simulink model "Reg_Adapt_c"  (R2017a)
settings: Solver=ode1  StartTime=0.0  StopTime=10  FixedStep=0.0001  RelTol=1e-3
values from neighbouring files (symbols this model uses):
  gamma = 0.005    [Dane_reg_adapt.m]
  Kd1 = 0.09    [Dane_reg_adapt.m]
  Ki1 = 350    [Dane_reg_adapt.m]
  Kp1 = 7    [Dane_reg_adapt.m]
  ksi = 0.9    [Dane_reg_adapt.m]
  omega = 40    [Dane_reg_adapt.m]
  Te = 0.001    [Dane_reg_adapt.m]
  Tm = 0.2    [Dane_reg_adapt.m]
  W1init = -1*0.1    (= -0.1)    [Dane_reg_adapt.m]
  W2init = 0.2    [Dane_reg_adapt.m]
  W3init = 0.3    [Dane_reg_adapt.m]
  W4init = -1*0.4    (= -0.4)    [Dane_reg_adapt.m]
  W5init = -1*0.5    (= -0.5)    [Dane_reg_adapt.m]
  W6init = 0.6    [Dane_reg_adapt.m]
libraries: neural x6
settings Model: Creator=kamil  LastModifiedBy=kamil

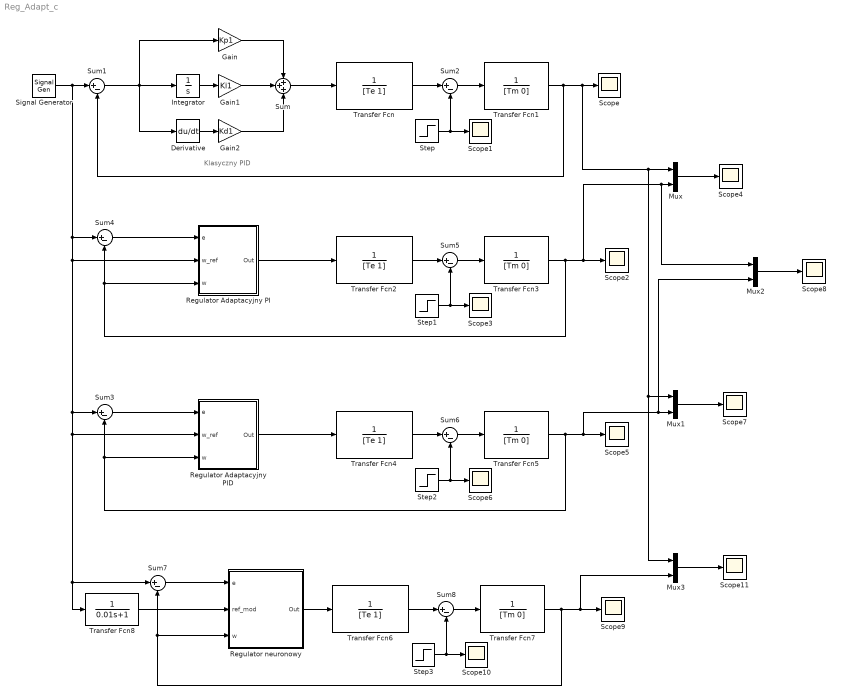
== system Reg_Adapt_c ==
  note: Klasyczny PID
  Derivative : Derivative
  Gain : Gain  Gain=Kp1
  Gain1 : Gain  Gain=Ki1
  Gain2 : Gain  Gain=Kd1
  Integrator : Integrator
  Mux{,1..3} (4 alike) : Mux  Inputs=2
  Regulator Adaptacyjny PI : Subsystem
  Regulator Adaptacyjny PID : Subsystem
  Regulator neuronowy : Subsystem
  Scope{,1..11} (12 alike) : Scope
  Signal Generator : SignalGenerator  WaveForm=square
  Step : Step  Time=2.25  SampleTime=0
  Step1 : Step  SampleTime=0
  Step2 : Step  SampleTime=0
  Step3 : Step  SampleTime=0
  Sum : Sum  Inputs=+++
  Sum{1..8} (8 alike) : Sum  Inputs=|+-
  Transfer Fcn{,2,4,6} (4 alike) : TransferFcn  Denominator=[Te 1]
  Transfer Fcn{1,3,5,7} (4 alike) : TransferFcn  Denominator=[Tm 0]
  Transfer Fcn8 : TransferFcn  Denominator=[0.01 1]
  wires:
  Gain/1 -> Sum/1
  Gain1/1 -> Sum/2
  Gain2/1 -> Sum/3
  Sum1/1 -> Integrator/1, Gain/1, Derivative/1
  Sum/1 -> Transfer Fcn/1
  Sum2/1 -> Transfer Fcn1/1
  Transfer Fcn/1 -> Sum2/1
  Step/1 -> Scope1/1, Sum2/2
  Integrator/1 -> Gain1/1
  Derivative/1 -> Gain2/1
  Sum4/1 -> Regulator Adaptacyjny PI/1(e)
  Step1/1 -> Scope3/1, Sum5/2
  Regulator Adaptacyjny PI/1(Out) -> Transfer Fcn2/1
  Sum5/1 -> Transfer Fcn3/1
  Transfer Fcn2/1 -> Sum5/1
  Mux/1 -> Scope4/1
  Transfer Fcn4/1 -> Sum6/1
  Sum3/1 -> Regulator Adaptacyjny PID/1(e)
  Sum6/1 -> Transfer Fcn5/1
  Step2/1 -> Scope6/1, Sum6/2
  Regulator Adaptacyjny PID/1(Out) -> Transfer Fcn4/1
  Mux1/1 -> Scope7/1
  Transfer Fcn5/1 -> Mux2/2, Mux1/2, Scope5/1, Regulator Adaptacyjny PID/3(w), Sum3/2
  Transfer Fcn3/1 -> Mux2/1, Mux/2, Scope2/1, Regulator Adaptacyjny PI/3(w), Sum4/2
  Mux2/1 -> Scope8/1
  Step3/1 -> Scope10/1, Sum8/2
  Regulator neuronowy/1(Out) -> Transfer Fcn6/1
  Transfer Fcn6/1 -> Sum8/1
  Signal Generator/1 -> Regulator Adaptacyjny PI/2(w_ref), Transfer Fcn8/1, Sum7/1, Regulator Adaptacyjny PID/2(w_ref), Sum3/1, Sum4/1, Sum1/1
  Sum8/1 -> Transfer Fcn7/1
  Sum7/1 -> Regulator neuronowy/1(e)
  Transfer Fcn1/1 -> Mux3/1, Mux1/1, Mux/1, Scope/1, Sum1/2
  Mux3/1 -> Scope11/1
  Transfer Fcn7/1 -> Mux3/2, Scope9/1, Sum7/2, Regulator neuronowy/3(w)
  Transfer Fcn8/1 -> Regulator neuronowy/2(ref_mod)

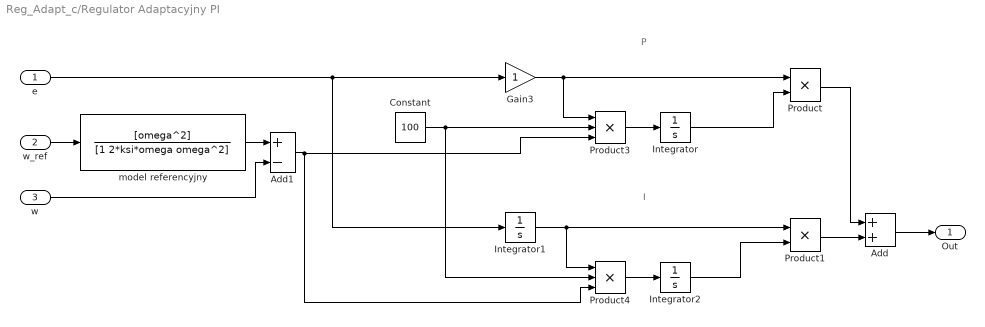
== system Reg_Adapt_c/Regulator Adaptacyjny PI ==
  note: P
  note: I
  e : Inport
  w_ref : Inport  Port=2
  w : Inport  Port=3
  Add : Sum
  Add1 : Sum  Inputs=+-
  Constant : Constant  Value=100
  Gain3 : Gain
  Integrator : Integrator  InitialCondition=Kp1
  Integrator1 : Integrator
  Integrator2 : Integrator  InitialCondition=Ki1
  Product : Product
  Product1 : Product
  Product3 : Product  Inputs=3
  Product4 : Product  Inputs=3
  model referencyjny : TransferFcn  Numerator=[omega^2]  Denominator=[1 2*ksi*omega omega^2]
  Out : Outport
  wires:
  Product1/1 -> Add/2
  e/1 -> Integrator1/1, Gain3/1
  Gain3/1 -> Product3/1, Product/1
  Product/1 -> Add/1
  Add1/1 -> Product4/3, Product3/3
  w_ref/1 -> model referencyjny/1
  w/1 -> Add1/2
  model referencyjny/1 -> Add1/1
  Add/1 -> Out/1
  Integrator2/1 -> Product1/2
  Product4/1 -> Integrator2/1
  Integrator1/1 -> Product4/1, Product1/1
  Constant/1 -> Product4/2, Product3/2
  Product3/1 -> Integrator/1
  Integrator/1 -> Product/2

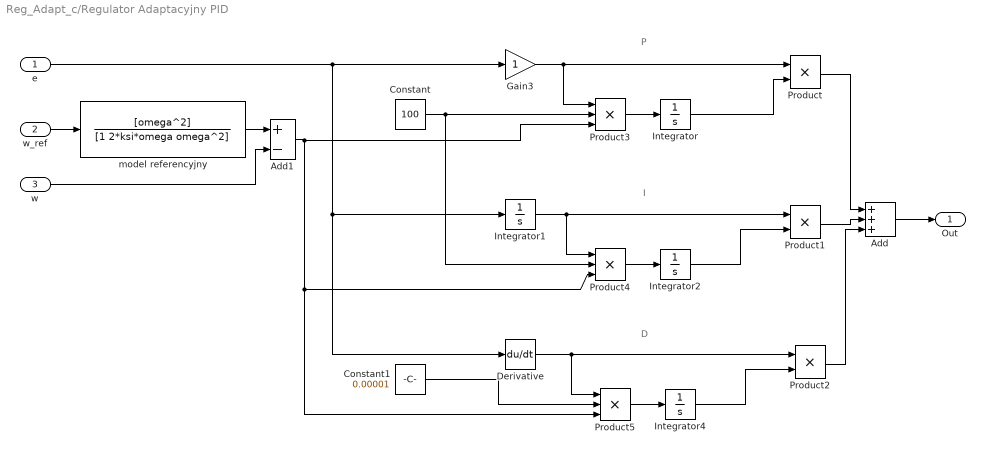
== system Reg_Adapt_c/Regulator Adaptacyjny PID ==
  note: P
  note: I
  note: D
  e : Inport
  w_ref : Inport  Port=2
  w : Inport  Port=3
  Add : Sum  Inputs=+++
  Add1 : Sum  Inputs=+-
  Constant : Constant  Value=100
  Constant1 : Constant  Value=0.00001
  Derivative : Derivative
  Gain3 : Gain
  Integrator : Integrator  InitialCondition=Kp1
  Integrator1 : Integrator
  Integrator2 : Integrator  InitialCondition=Ki1
  Integrator4 : Integrator  InitialCondition=Kd1
  Product : Product
  Product1 : Product
  Product2 : Product
  Product3 : Product  Inputs=3
  Product4 : Product  Inputs=3
  Product5 : Product  Inputs=3
  model referencyjny : TransferFcn  Numerator=[omega^2]  Denominator=[1 2*ksi*omega omega^2]
  Out : Outport
  wires:
  Product1/1 -> Add/2
  Gain3/1 -> Product3/1, Product/1
  Product/1 -> Add/1
  w_ref/1 -> model referencyjny/1
  w/1 -> Add1/2
  model referencyjny/1 -> Add1/1
  Add/1 -> Out/1
  Integrator2/1 -> Product1/2
  Product4/1 -> Integrator2/1
  Integrator1/1 -> Product4/1, Product1/1
  Product3/1 -> Integrator/1
  Integrator/1 -> Product/2
  e/1 -> Derivative/1, Integrator1/1, Gain3/1
  Derivative/1 -> Product5/1, Product2/1
  Constant/1 -> Product4/2, Product3/2
  Integrator4/1 -> Product2/2
  Product2/1 -> Add/3
  Add1/1 -> Product5/3, Product4/3, Product3/3
  Product5/1 -> Integrator4/1
  Constant1/1 -> Product5/2

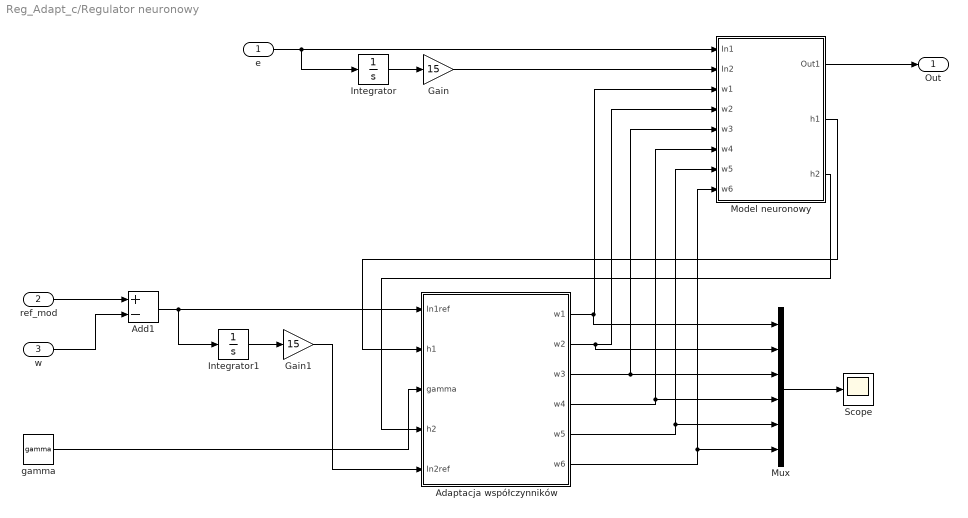
== system Reg_Adapt_c/Regulator neuronowy ==
  e : Inport
  ref_mod : Inport  Port=2
  w : Inport  Port=3
  Adaptacja współczynników : Subsystem
  Add1 : Sum  Inputs=+-
  Gain : Gain  Gain=15
  Gain1 : Gain  Gain=15
  Integrator : Integrator
  Integrator1 : Integrator
  Model neuronowy : Subsystem
  Mux : Mux  Inputs=6
  Scope : Scope
  gamma : Constant  Value=gamma
  Out : Outport
  wires:
  Adaptacja współczynników/6(w6) -> Mux/6, Model neuronowy/8(w6)
  gamma/1 -> Adaptacja współczynników/3(gamma)
  Mux/1 -> Scope/1
  Model neuronowy/2(h1) -> Adaptacja współczynników/2(h1)
  Adaptacja współczynników/5(w5) -> Mux/5, Model neuronowy/7(w5)
  Integrator1/1 -> Gain1/1
  Add1/1 -> Integrator1/1, Adaptacja współczynników/1(In1ref)
  Gain1/1 -> Adaptacja współczynników/5(In2ref)
  Gain/1 -> Model neuronowy/2(In2)
  Adaptacja współczynników/3(w3) -> Mux/3, Model neuronowy/5(w3)
  ref_mod/1 -> Add1/1
  Adaptacja współczynników/4(w4) -> Mux/4, Model neuronowy/6(w4)
  Adaptacja współczynników/1(w1) -> Mux/1, Model neuronowy/3(w1)
  Adaptacja współczynników/2(w2) -> Mux/2, Model neuronowy/4(w2)
  Model neuronowy/3(h2) -> Adaptacja współczynników/4(h2)
  w/1 -> Add1/2
  e/1 -> Integrator/1, Model neuronowy/1(In1)
  Integrator/1 -> Gain/1
  Model neuronowy/1(Out1) -> Out/1

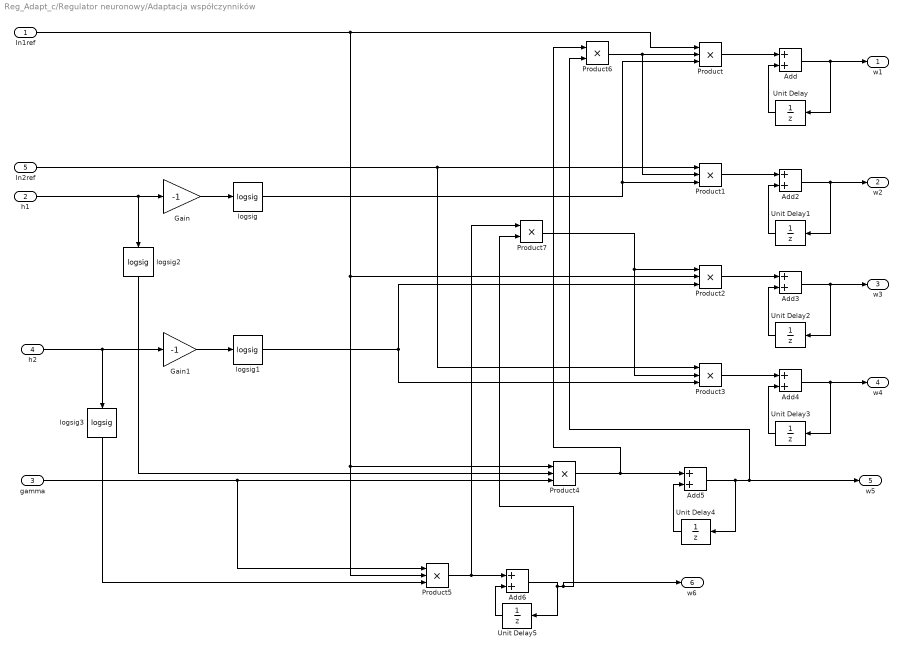
== system Reg_Adapt_c/Regulator neuronowy/Adaptacja współczynników ==
  In1ref : Inport
  h1 : Inport  Port=2
  gamma : Inport  Port=3
  h2 : Inport  Port=4
  In2ref : Inport  Port=5
  Add{,2..6} (6 alike) : Sum
  Gain : Gain  Gain=-1
  Gain1 : Gain  Gain=-1
  Product{,1..5} (6 alike) : Product  Inputs=3
  Product6 : Product
  Product7 : Product
  Unit Delay : UnitDelay  InitialCondition=W1init  SampleTime=-1
  Unit Delay1 : UnitDelay  InitialCondition=W2init  SampleTime=-1
  Unit Delay2 : UnitDelay  InitialCondition=W3init  SampleTime=-1
  Unit Delay3 : UnitDelay  InitialCondition=W4init  SampleTime=-1
  Unit Delay4 : UnitDelay  InitialCondition=W5init  SampleTime=-1
  Unit Delay5 : UnitDelay  InitialCondition=W6init  SampleTime=-1
  logsig{,1..3} (4 alike) : neural/Transfer Functions/logsig
      settings: SourceProductName=Neural Network Toolbox  SourceProductBaseCode=NN
  w1 : Outport
  w2 : Outport  Port=2
  w3 : Outport  Port=3
  w4 : Outport  Port=4
  w5 : Outport  Port=5
  w6 : Outport  Port=6
  wires:
  Product7/1 -> Product3/2, Product2/1
  Gain/1 -> logsig/1
  h2/1 -> logsig3/1, Gain1/1
  logsig1/1 -> Product3/3, Product2/3
  In1ref/1 -> Product/1, Product2/2, Product4/1, Product5/2
  Unit Delay1/1 -> Add2/2
  Unit Delay3/1 -> Add4/2
  Product2/1 -> Add3/1
  Unit Delay/1 -> Add/2
  Add/1 -> w1/1, Unit Delay/1
  Product/1 -> Add/1
  Add4/1 -> w4/1, Unit Delay3/1
  Add5/1 -> w5/1, Product6/2, Unit Delay4/1
  Product5/1 -> Product7/1, Add6/1
  Unit Delay5/1 -> Add6/2
  Add3/1 -> w3/1, Unit Delay2/1
  Product6/1 -> Product1/2, Product/2
  Unit Delay2/1 -> Add3/2
  Add2/1 -> w2/1, Unit Delay1/1
  gamma/1 -> Product5/1, Product4/3
  Add6/1 -> w6/1, Product7/2, Unit Delay5/1
  Unit Delay4/1 -> Add5/2
  Product1/1 -> Add2/1
  Product4/1 -> Product6/1, Add5/1
  Product3/1 -> Add4/1
  Gain1/1 -> logsig1/1
  logsig2/1 -> Product4/2
  logsig3/1 -> Product5/3
  In2ref/1 -> Product3/1, Product1/1
  logsig/1 -> Product1/3, Product/3
  h1/1 -> logsig2/1, Gain/1

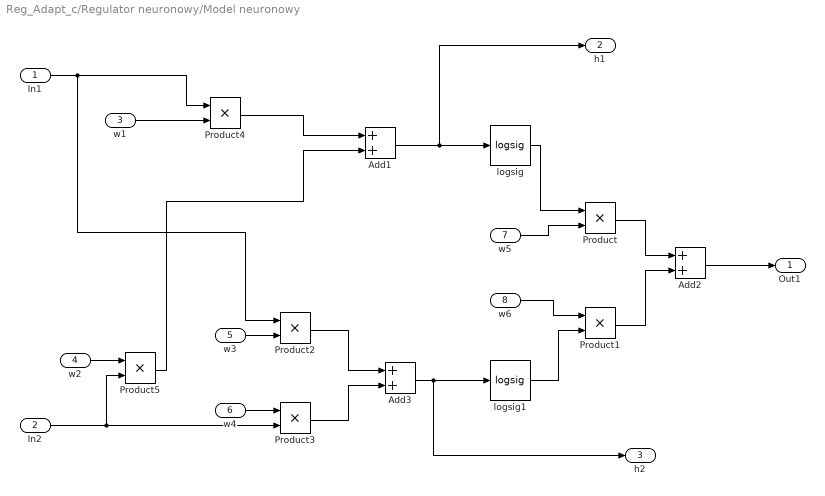
== system Reg_Adapt_c/Regulator neuronowy/Model neuronowy ==
  In1 : Inport
  In2 : Inport  Port=2
  w1 : Inport  Port=3
  w2 : Inport  Port=4
  w3 : Inport  Port=5
  w4 : Inport  Port=6
  w5 : Inport  Port=7
  w6 : Inport  Port=8
  Add1 : Sum
  Add2 : Sum
  Add3 : Sum
  Product{,1..5} (6 alike) : Product
  logsig : neural/Transfer Functions/logsig
      settings: SourceProductName=Neural Network Toolbox  SourceProductBaseCode=NN
  logsig1 : neural/Transfer Functions/logsig
      settings: SourceProductName=Neural Network Toolbox  SourceProductBaseCode=NN
  Out1 : Outport
  h1 : Outport  Port=2
  h2 : Outport  Port=3
  wires:
  Add1/1 -> h1/1, logsig/1
  Product1/1 -> Add2/2
  w4/1 -> Product3/1
  Add3/1 -> h2/1, logsig1/1
  w6/1 -> Product1/1
  w3/1 -> Product2/2
  In1/1 -> Product2/1, Product4/1
  w1/1 -> Product4/2
  w2/1 -> Product5/1
  In2/1 -> Product5/2, Product3/2
  Product4/1 -> Add1/1
  Add2/1 -> Out1/1
  Product3/1 -> Add3/2
  Product2/1 -> Add3/1
  logsig/1 -> Product/1
  Product5/1 -> Add1/2
  logsig1/1 -> Product1/2
  w5/1 -> Product/2
  Product/1 -> Add2/1
